simulink model "Linearhopf_squaretorque_0_5"  (R2019b)
settings: Solver=ode45  StartTime=0.0  StopTime=10  MaxStep=1e-3  RelTol=1e-3  AbsTol=1e-3
model workspace: external: MATLAB File sm_bumper_car_parameters.m (data not in the file)
undefined symbols (not defined in the file): BackLeft, BackRight, car, critical_velocity, damping, FrontLeft, FrontRight, g, kinetic_friction_coef, Link1, Link2, Link3, Link4, Link5, Link6, Link7, Link8, Link9, static_friction_coef, stiffness, transition_region_width, Wheel5, Wheel6, Wheel7, Wheel8, Wheel9, X, Y, Z
libraries: sm_lib x74, nesl_utility x19, sm_bumper_car_lib x9, simulink x7
(part 1 of 2)
Description:
  | Using the Spatial Contact Force Block - Bumper Car
settings Model: Creator=MathWorks  LastModifiedBy=hellomisscao
settings SolverCC: AutoScaleAbsTol=off
settings DataIOCC: ReturnWorkspaceOutputs=off
settings DebuggingCC: SymbolicDimsDataTypeCodeGenerationDiagnostic=none
settings SimscapeCC: SimscapeLogType=all  SimscapeLogSimulationStatistics=on  SimscapeLogName=simlog_sm_bumper_car  SimscapeLogDataHistory=20000
settings ExplorerConfigSet: InternalSimMechanicsExplorerSettings="<ExplorerConfiguration><canonicalview>default</canonicalview><AnimationSetting><BasePlaybackSpeed>1.0</BasePlaybackSpeed><PlaybackSpeedFactor>1.0</PlaybackSpeedFactor></AnimationSetting><TilePanel><TileInfo><Tiles Columns=\"1\" Count=\"1\" Rows=\"1\"><Column Weight=\"1\"/><Row Weight=\"1\"/><Tile Height=\"1\" Width=\"1\" X=\"0\" Y=\"0\"/></Tiles></TileInfo><SceneInfo><SceneViewer><BGColor><R>0.800000011920928955</R><G>0.800000011920928955</G><B>0.800000011920928955</B></BGColor><Camera><DoPerspective>off</DoPerspective><Position><X>0.637508295609907183</X><Y>-0.637508296451667844</Y><Z>1.11601012334107264</Z></Position><Center><X>-0.00639254054797280813</X><Y>0.00639253970621195267</Y><Z>0.472109287183192672</Z></Center><Up><X>-0.408248290463863073</X><Y>0.408248290463863073</Y><Z>0.816496580927726145</Z></Up><ViewLimDist>1</ViewLimDist><YLim>0.759088869094848628</YLim><XLim>0.995304530142192112</XLim></Camera></SceneViewer></SceneInfo></TilePanel><MechEditorPanel><Cameras/><GfxPanelCameraMap/><VideoCreator><PlaybackSpeedRatio>1.0</PlaybackSpeedRatio><FrameRate>30</FrameRate><VideoFormat>Motion JPEG AVI</VideoFormat><FrameSize>auto</FrameSize></VideoCreator></MechEditorPanel></ExplorerConfiguration>"

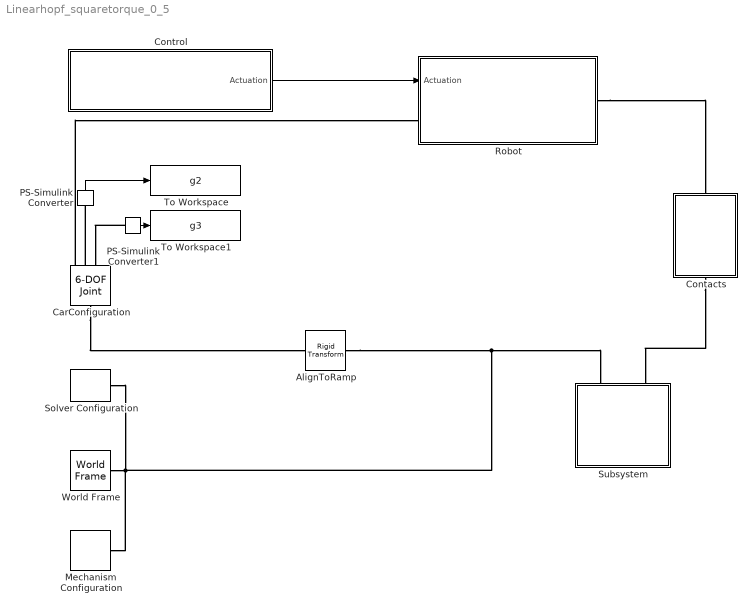
== system Linearhopf_squaretorque_0_5 ==
  AlignToRamp : sm_lib/Frames and Transforms/Rigid Transform  TranslationMethod=StandardAxis  TranslationStandardOffset=50 + 2*car.wheel.radius + 1  TranslationLengthUnit=cm  TranslationStandardAxis=+Z  TranslationCartesianOffset=[0 0 0]  TranslationROffset=0  TranslationROffsetUnits=m  TranslationZOffset=0  TranslationZOffsetUnits=m  TranslationThetaOffset=0  TranslationThetaOffsetUnits=deg  RotationMethod=StandardAxis  RotationAngleUnits=deg  RotationStandardAxis=+Y  RotationAngle=0  RotationArbitraryAxis=[0 0 1]  FollAlignAxisA=+X  BaseAlignAxisA=+Y  FollAlignAxisB=+Y  BaseAlignAxisB=+Z  RotationSequenceAxes=FollowerAxes  RotationSequence=XYX  RotationSequenceAngles=[0 0 0]  RotationSequenceAnglesUnits=deg  RotationMatrix=[1 0 0; 0 1 0; 0 0 1]
  CarConfiguration : sm_lib/Joints/6-DOF Joint  JointMode=Normal  SenseConstraintForce=off  SenseConstraintForceX=off  SenseConstraintForceY=off  SenseConstraintForceZ=off  SenseConstraintTorque=off  SenseConstraintTorqueX=off  SenseConstraintTorqueY=off  SenseConstraintTorqueZ=off  SenseTotalForce=off  SenseTotalForceX=off  SenseTotalForceY=off  SenseTotalForceZ=off  SenseTotalTorque=off  SenseTotalTorqueX=off  SenseTotalTorqueY=off  SenseTotalTorqueZ=off  CompositeWrenchDir=FollowerOnBase  CompositeWrenchFrame=BaseFrame  PxEquilibriumPosition=0  PxEquilibriumPositionUnits=m  PxSpringStiffness=0  PxSpringStiffnessUnits=N/m  PxDampingCoefficient=0  PxDampingCoefficientUnits=N/(m/s)  PxTorqueActuationMode=NoTorque  PxMotionActuationMode=ComputedMotion  PxSensePosition=on  PxSenseVelocity=off  PxSenseAcceleration=off  PxSenseTorqueForce=off  PxSenseLowerLimitTorqueForce=off  PxSenseUpperLimitTorqueForce=off  PxLowerLimitSpecify=off  PxLowerLimitBound=-1  PxLowerLimitBoundUnits=m  PxLowerLimitStiffness=1e6  PxLowerLimitStiffnessUnits=N/m  PxLowerLimitDamping=1e3  PxLowerLimitDampingUnits=N/(m/s)  PxLowerLimitTransitionRegionWidth=1e-4  PxLowerLimitTransitionRegionWidthUnits=m  PxUpperLimitSpecify=off  PxUpperLimitBound=1  PxUpperLimitBoundUnits=m  PxUpperLimitStiffness=1e6  PxUpperLimitStiffnessUnits=N/m  PxUpperLimitDamping=1e3  PxUpperLimitDampingUnits=N/(m/s)  PxUpperLimitTransitionRegionWidth=1e-4  PxUpperLimitTransitionRegionWidthUnits=m  PxPositionTargetSpecify=on  PxPositionTargetPriority=High  PxPositionTargetValue=car.start_dist  PxPositionTargetValueUnits=cm  PxVelocityTargetSpecify=off  PxVelocityTargetPriority=High  PxVelocityTargetValue=0  PxVelocityTargetValueUnits=m/s  PyEquilibriumPosition=0  PyEquilibriumPositionUnits=m  PySpringStiffness=0  PySpringStiffnessUnits=N/m  PyDampingCoefficient=0  PyDampingCoefficientUnits=N/(m/s)  PyTorqueActuationMode=NoTorque  PyMotionActuationMode=ComputedMotion  PySensePosition=on  PySenseVelocity=off  PySenseAcceleration=off  PySenseTorqueForce=off  PySenseLowerLimitTorqueForce=off  PySenseUpperLimitTorqueForce=off  PyLowerLimitSpecify=off  PyLowerLimitBound=-1  PyLowerLimitBoundUnits=m  PyLowerLimitStiffness=1e6  PyLowerLimitStiffnessUnits=N/m  PyLowerLimitDamping=1e3  PyLowerLimitDampingUnits=N/(m/s)  PyLowerLimitTransitionRegionWidth=1e-4  PyLowerLimitTransitionRegionWidthUnits=m  PyUpperLimitSpecify=off  PyUpperLimitBound=1  PyUpperLimitBoundUnits=m  PyUpperLimitStiffness=1e6  PyUpperLimitStiffnessUnits=N/m  PyUpperLimitDamping=1e3  PyUpperLimitDampingUnits=N/(m/s)  PyUpperLimitTransitionRegionWidth=1e-4  PyUpperLimitTransitionRegionWidthUnits=m  PyPositionTargetSpecify=off  PyPositionTargetPriority=High  PyPositionTargetValue=0  PyPositionTargetValueUnits=m  PyVelocityTargetSpecify=off  PyVelocityTargetPriority=High  PyVelocityTargetValue=0  PyVelocityTargetValueUnits=m/s  PzEquilibriumPosition=0  PzEquilibriumPositionUnits=m  PzSpringStiffness=0  PzSpringStiffnessUnits=N/m  PzDampingCoefficient=0  PzDampingCoefficientUnits=N/(m/s)  PzTorqueActuationMode=NoTorque  PzMotionActuationMode=ComputedMotion  PzSensePosition=on  PzSenseVelocity=off  PzSenseAcceleration=off  PzSenseTorqueForce=off  PzSenseLowerLimitTorqueForce=off  PzSenseUpperLimitTorqueForce=off  PzLowerLimitSpecify=off  PzLowerLimitBound=-1  PzLowerLimitBoundUnits=m  PzLowerLimitStiffness=1e6  PzLowerLimitStiffnessUnits=N/m  PzLowerLimitDamping=1e3  PzLowerLimitDampingUnits=N/(m/s)  PzLowerLimitTransitionRegionWidth=1e-4  PzLowerLimitTransitionRegionWidthUnits=m  PzUpperLimitSpecify=off  PzUpperLimitBound=1  PzUpperLimitBoundUnits=m  PzUpperLimitStiffness=1e6  PzUpperLimitStiffnessUnits=N/m  PzUpperLimitDamping=1e3  PzUpperLimitDampingUnits=N/(m/s)  PzUpperLimitTransitionRegionWidth=1e-4  PzUpperLimitTransitionRegionWidthUnits=m  PzPositionTargetSpecify=on  PzPositionTargetPriority=High  PzPositionTargetValue=car.start_height  PzPositionTargetValueUnits=cm  PzVelocityTargetSpecify=off  PzVelocityTargetPriority=High  PzVelocityTargetValue=0  PzVelocityTargetValueUnits=m/s  SphDefPosRotationMethod=None  SphDefPosRotationAngleUnits=deg  SphDefPosRotationStandardAxis=+Z  SphDefPosRotationAngle=0.0  SphDefPosRotationArbitraryAxis=[0 0 1]  SphDefPosFollAlignAxisA=+X  SphDefPosBaseAlignAxisA=+Y  SphDefPosFollAlignAxisB=+Y  SphDefPosBaseAlignAxisB=+Z  SphDefPosRotationSequenceAxes=FollowerAxes  SphDefPosRotationSequence=XYX  SphDefPosRotationSequenceAngles=[0 0 0]  SphDefPosRotationSequenceAnglesUnits=deg  SphDefPosRotationMatrix=[1 0 0; 0 1 0; 0 0 1]  SphEqPosRotationMethod=None  SphEqPosRotationAngleUnits=deg  SphEqPosRotationStandardAxis=+Z  SphEqPosRotationAngle=0.0  SphEqPosRotationArbitraryAxis=[0 0 1]  SphEqPosFollAlignAxisA=+X  SphEqPosBaseAlignAxisA=+Y  SphEqPosFollAlignAxisB=+Y  SphEqPosBaseAlignAxisB=+Z  SphEqPosRotationSequenceAxes=FollowerAxes  SphEqPosRotationSequence=XYX  SphEqPosRotationSequenceAngles=[0 0 0]  SphEqPosRotationSequenceAnglesUnits=deg  SphEqPosRotationMatrix=[1 0 0; 0 1 0; 0 0 1]  SphSpringStiffness=0  SphSpringStiffnessUnits=N*m/deg  SphDampingCoefficient=0  SphDampingCoefficientUnits=N*m/(deg/s)  SphActuateTorqueX=off  SphActuateTorqueY=off  SphActuateTorqueZ=off  SphActuateTorque=off  SphTorqueActuationMode=NoTorque  SphMotionActuationMode=ComputedMotion  SphActuationFrame=BaseFrame  SphSensePosition=off  SphSenseVelocityX=off  SphSenseVelocityY=off  SphSenseVelocityZ=off  SphSenseVelocity=off  SphSenseAccelerationX=off  SphSenseAccelerationY=off  SphSenseAccelerationZ=off  SphSenseAcceleration=off  SphSenseTorqueX=off  SphSenseTorqueY=off  SphSenseTorqueZ=off  SphSenseTorqueForce=off  SphSenseLowerLimitTorqueMag=off  SphSenseUpperLimitTorqueMag=off  SphSensingFrame=BaseFrame  SphLowerLimitSpecify=off  SphLowerLimitBound=15  SphLowerLimitBoundUnits=deg  SphLowerLimitStiffness=1e4  SphLowerLimitStiffnessUnits=N*m/deg  SphLowerLimitDamping=10  SphLowerLimitDampingUnits=N*m/(deg/s)  SphLowerLimitTransitionRegionWidth=0.1  SphLowerLimitTransitionRegionWidthUnits=deg  SphUpperLimitSpecify=off  SphUpperLimitBound=45  SphUpperLimitBoundUnits=deg  SphUpperLimitStiffness=1e4  SphUpperLimitStiffnessUnits=N*m/deg  SphUpperLimitDamping=10  SphUpperLimitDampingUnits=N*m/(deg/s)  SphUpperLimitTransitionRegionWidth=0.1  SphUpperLimitTransitionRegionWidthUnits=deg  SphPositionTargetRotationMethod=StandardAxis  SphPositionTargetRotationAngleUnits=deg  SphPositionTargetRotationStandardAxis=-Y  SphPositionTargetRotationAngle=car.start_pitch  SphPositionTargetRotationArbitraryAxis=[0 0 1]  SphPositionTargetFollAlignAxisA=+X  SphPositionTargetBaseAlignAxisA=+Y  SphPositionTargetFollAlignAxisB=+Y  SphPositionTargetBaseAlignAxisB=+Z  SphPositionTargetRotationSequenceAxes=FollowerAxes  SphPositionTargetRotationSequence=XYX  SphPositionTargetRotationSequenceAngles=[0 0 0]  SphPositionTargetRotationSequenceAnglesUnits=deg  SphPositionTargetRotationMatrix=[1 0 0; 0 1 0; 0 0 1]  SphPositionTargetSpecify=off  SphPositionTargetPriority=High  SphVelocityTargetValue=[0 0 0]  SphVelocityTargetValueUnits=deg/s  SphVelocityTargetSpecify=off  SphVelocityTargetPriority=High  SphVelocityTargetInFollowerFrame=on
  Contacts : Subsystem  mask{k=stiffness, b=damping, tau=transition_region_width, mus=static_friction_coef, muk=kinetic_friction_coef, cv=critical_velocity}
      mask prompts: k "Stiffness (N/m)"; b "Damping (N/(m/s))"; tau "Transition Region Width (m)"; mus "Coefficient of Static Friction"; muk "Coefficient of Kinetic Friction"; cv "Critical Velocity (m/s)"
  Control : Subsystem
  Mechanism Configuration : sm_lib/Utilities/Mechanism Configuration  UniformGravity=Constant  GravityVector=[0 0 -g]  GravityUnits=m/s^2  LinearizationDelta=0.001
  PS-Simulink Converter : nesl_utility/PS-Simulink Converter  PhysicalDomain=network_engine_domain  SubClassName=ps_output  LeftPortType=input  RightPortType=output  PseudoPeriodic=off  Frequencies=[]  Unit=inherit  AffineConversion=off
  PS-Simulink Converter1 : nesl_utility/PS-Simulink Converter  PhysicalDomain=network_engine_domain  SubClassName=ps_output  LeftPortType=input  RightPortType=output  PseudoPeriodic=off  Frequencies=[]  Unit=inherit  AffineConversion=off
  Robot : Subsystem  mask{l=car.body.length, w=car.body.width, h=car.body.height, m=car.body.mass, body_color=car.body.color, wheel_radius=car.wheel.radius, wheel_width=car.wheel.thickness, wheel_m=car.wheel.mass, wheel_color=car.wheel.color, wheel_spoke_color=car.wheel.spoke.color}
      mask prompts: l "Length (cm)"; w "Width (cm)"; h "Height (cm)"; m "Body Mass (kg)"; body_color "Car Body Color"; wheel_radius "Radius"; wheel_width "Thickness"; wheel_m "Wheel Mass (kg)"; wheel_color "Wheel Color"; wheel_spoke_color "Wheel Spoke Color"
      mask init:
      | axle_len               = .85 * l;
      | axle_radius            = axle_len / 30;
      | wheel_inner_radius     = .67 * wheel_radius;
      | wheel_spoke_thickness = axle_radius / 2;
      | 
      | front_wheel_pos  = l * .12;
      | back_wheel_pos   = l * .88;
      | wheel_separation = axle_len;
      mask DialogControl BodyGroupVar Prompt: Body
      mask DialogControl BodyDimGroupVar Prompt: Dimensions
      mask DialogControl BodyInertiaGroupVar Prompt: Inertia
      mask DialogControl BodyGraphicGroupVar Prompt: Graphic
      mask DialogControl WheelGroupVar Prompt: Wheels
      mask DialogControl WheelDimGroupVar Prompt: Dimensions
      mask DialogControl WheelInertiaGroupVar Prompt: Inertia
      mask DialogControl WheelGraphicGroupVar Prompt: Graphic
      mask Display: image('$imagefile'); % Use "Edit Image" on toolstrip to change.
  Solver Configuration : nesl_utility/Solver Configuration  PhysicalDomain=network_engine_domain  SubClassName=solver  LeftPortType=input  RightPortType=generic  Tones=[]  Harmonics=[]  SimulateNoise=off  Profile=off  UseLocalSampling=off  EnableSwitchedLinearOptims=on  FrequencyDomain=off  UseCCode=off  RelTol=0.001  AbsTol=1e-06  MinStep=1e-09  ToWorkspace=off  RevertToSquareIcSolve=off  NumHomotopyIterations=100  PhasorMode=off  PhasorModeNumHarmonics=1  DoDC=off  ResidualTolerance=1e-09  UseLocalSolver=off  LocalSolverChoice=NE_BACKWARD_EULER_ADVANCER  LocalSolverSampleTime=0.001  DoFixedCost=off  MaxNonlinIter=3  MaxModeIter=2  LinearAlgebra=Sparse  EquationFormulation=NE_TIME_EF  DelaysMemoryBudget=1024  AutomaticFiltering=on  FilteringTimeConstant=0.001  PartitionStorageMethod=AS_NEEDED  PartitionMemoryBudget=1024  PartitionMethod=FAST
  Subsystem : Subsystem
  To Workspace : ToWorkspace  VariableName=g2  SampleTime=-1
  To Workspace1 : ToWorkspace  VariableName=g3  SampleTime=-1
  World Frame : sm_lib/Frames and Transforms/World Frame
  wires:
  Control/1(Actuation) -> Robot/1(Actuation)
  PS-Simulink Converter/1 -> To Workspace/1
  PS-Simulink Converter1/1 -> To Workspace1/1
  connections:
  CarConfiguration/RConn1 -- Robot/LConn1
  Solver Configuration/RConn1 -- Mechanism Configuration/RConn1 -- Subsystem/RConn1 -- AlignToRamp/LConn1 -- World Frame/RConn1
  Robot/RConn1 -- Contacts/RConn1
  Contacts/LConn1 -- Subsystem/RConn2
  CarConfiguration/LConn1 -- AlignToRamp/RConn1
  CarConfiguration/RConn2 -- PS-Simulink Converter/LConn1
  PS-Simulink Converter1/LConn1 -- CarConfiguration/RConn3

== system Linearhopf_squaretorque_0_5/Contacts ==
  Car to Ramp 1 : Subsystem
  Ramps : PMIOPort  Side=Left
  Car : PMIOPort  Port=2  Side=Right
  connections:
  Car/RConn1 -- Car to Ramp 1/RConn1
  Ramps/RConn1 -- Car to Ramp 1/LConn1

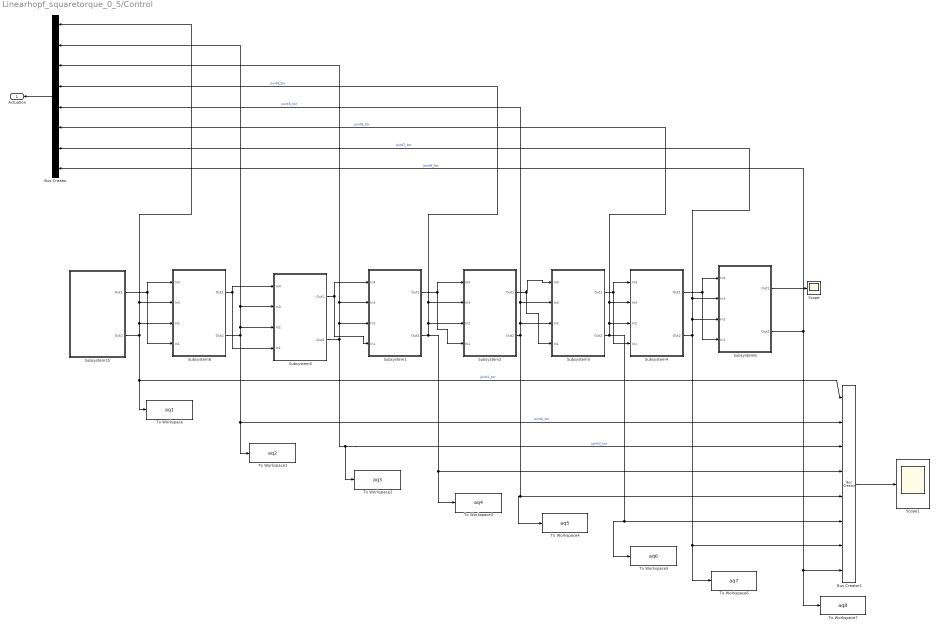
== system Linearhopf_squaretorque_0_5/Control ==
  Bus Creator : BusCreator  Inputs=8
  Bus Creator1 : BusCreator  Inputs=8
  Scope : Scope
  Scope1 : Scope
  Subsystem1 : Subsystem
  Subsystem15 : Subsystem
  Subsystem2 : Subsystem
  Subsystem3 : Subsystem
  Subsystem4 : Subsystem
  Subsystem5 : Subsystem
  Subsystem6 : Subsystem
  Subsystem8 : Subsystem
  To Workspace : ToWorkspace  VariableName=aq1  SaveFormat=Timeseries  SampleTime=-1
  To Workspace1 : ToWorkspace  VariableName=aq2  SaveFormat=Timeseries  SampleTime=-1
  To Workspace2 : ToWorkspace  VariableName=aq3  SaveFormat=Timeseries  SampleTime=-1
  To Workspace3 : ToWorkspace  VariableName=aq4  SaveFormat=Timeseries  SampleTime=-1
  To Workspace4 : ToWorkspace  VariableName=aq5  SaveFormat=Timeseries  SampleTime=-1
  To Workspace5 : ToWorkspace  VariableName=aq6  SaveFormat=Timeseries  SampleTime=-1
  To Workspace6 : ToWorkspace  VariableName=aq7  SaveFormat=Timeseries  SampleTime=-1
  To Workspace7 : ToWorkspace  VariableName=aq8  SaveFormat=Timeseries  SampleTime=-1
  Actuation : Outport
  wires:
  Subsystem5/2(Out2) -> Subsystem1/3(In2), Subsystem1/2(In3), Bus Creator/3, Bus Creator1/3, To Workspace2/1  "joint3_tor"
  Subsystem3/2(Out2) -> Subsystem4/3(In2), Bus Creator/6, Subsystem4/2(In3), To Workspace5/1, Bus Creator1/6  "joint6_tor"
  Subsystem8/2(Out2) -> Bus Creator/2, Subsystem5/2(In3), Subsystem5/3(In2), Bus Creator1/2, To Workspace1/1  "joint2_tor"
  Bus Creator/1 -> Actuation/1
  Subsystem1/2(Out2) -> To Workspace3/1, Bus Creator1/4, Subsystem2/2(In3), Bus Creator/4, Subsystem2/3(In2)  "joint4_tor"
  Subsystem4/2(Out2) -> To Workspace6/1, Bus Creator1/7, Subsystem6/3(In2), Bus Creator/7, Subsystem6/2(In3)  "joint7_tor"
  Subsystem6/2(Out2) -> To Workspace7/1, Bus Creator1/8, Bus Creator/8  "joint8_tor"
  Subsystem2/2(Out2) -> Subsystem3/3(In2), Bus Creator/5, Subsystem3/2(In3), To Workspace4/1, Bus Creator1/5  "joint5_tor"
  Subsystem15/2(Out2) -> To Workspace/1, Bus Creator1/1, Subsystem8/2(In3), Bus Creator/1, Subsystem8/3(In2)  "joint1_tor"
  Subsystem4/1(Out1) -> Subsystem6/1(In4), Subsystem6/4(In1)
  Subsystem3/1(Out1) -> Subsystem4/1(In4), Subsystem4/4(In1)
  Subsystem15/1(Out1) -> Subsystem8/4(In1), Subsystem8/1(In4)
  Subsystem1/1(Out1) -> Subsystem2/4(In1), Subsystem2/1(In4)
  Subsystem6/1(Out1) -> Scope/1
  Bus Creator1/1 -> Scope1/1
  Subsystem8/1(Out1) -> Subsystem5/4(In1), Subsystem5/1(In4)
  Subsystem5/1(Out1) -> Subsystem1/1(In4), Subsystem1/4(In1)
  Subsystem2/1(Out1) -> Subsystem3/1(In4), Subsystem3/4(In1)

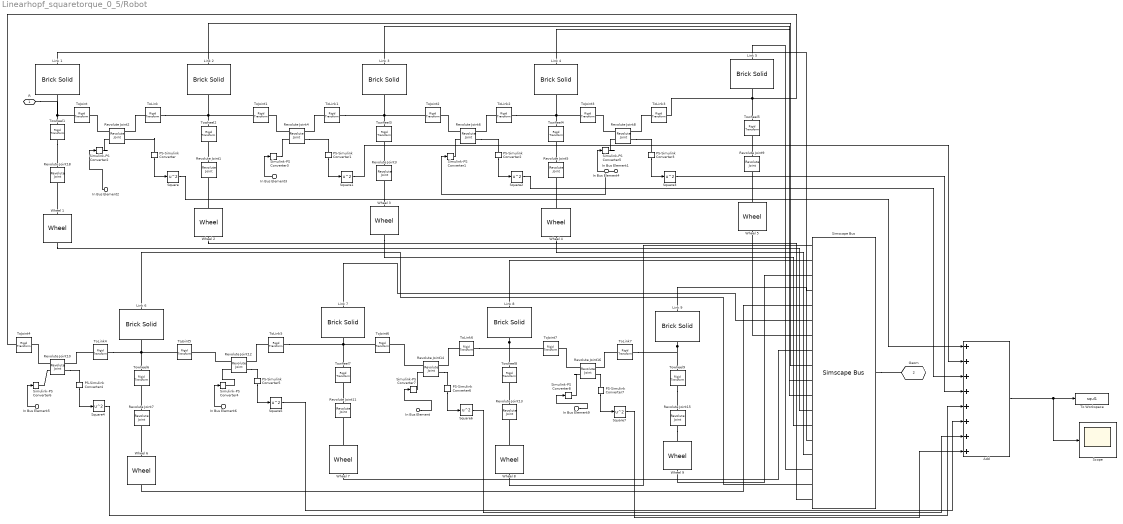
== system Linearhopf_squaretorque_0_5/Robot ==
  In Bus Element2 : Inport  PortName=Actuation  Element=joint1_tor
  In Bus Element3 : Inport  PortName=Actuation  Element=joint2_tor
  In Bus Element1 : Inport  PortName=Actuation  Element=joint3_tor
  In Bus Element4 : Inport  PortName=Actuation  Element=joint4_tor
  In Bus Element5 : Inport  PortName=Actuation  Element=joint5_tor
  In Bus Element6 : Inport  PortName=Actuation  Element=joint6_tor
  In Bus Element : Inport  PortName=Actuation  Element=joint7_tor
  In Bus Element9 : Inport  PortName=Actuation  Element=joint8_tor
  Add : Sum  Inputs=++++++++
  Link 1 : sm_lib/Body Elements/Brick Solid  GraphicAmbientColor=[0.15 0.15 0.15 1.0]  BasedOnType=Mass  BrickDimensions=[l w h]  BrickDimensionUnits=cm  CenterOfMass=[0 0 0]  CenterOfMassUnits=cm  GraphicDiffuseColor=[0.8 0.8 0.0]  Density=1000  DensityUnits=kg/m^3  DoExposeReferenceFrame=on  GraphicEmissiveColor=[0.0 0.0 0.0 1.0]  ExportEntireGeometry=on  SerializedFrames=<Frames/>  MarkerShape=Sphere  MarkerSize=10  GraphicType=FromGeometry  InertiaType=CalculateFromGeometry  Mass=m  MassUnits=kg  MomentsOfInertia=[1 1 1]  MomentsOfInertiaUnits=kg*m^2  GraphicOpacity=1.0  ProductsOfInertia=[0 0 0]  ProductsOfInertiaUnits=kg*m^2  GraphicShininess=75  GraphicSpecularColor=[0.5 0.5 0.5 1.0]  GraphicVisPropType=SimpleVisualProperties
  Link {2..9} (8 alike) : sm_lib/Body Elements/Brick Solid  GraphicAmbientColor=[0.15 0.15 0.15 1.0]  BasedOnType=Mass  BrickDimensions=[l w h]  BrickDimensionUnits=cm  CenterOfMass=[0 0 0]  CenterOfMassUnits=cm  GraphicDiffuseColor=[1.0 0.2 0.0]  Density=1000  DensityUnits=kg/m^3  DoExposeReferenceFrame=on  GraphicEmissiveColor=[0.0 0.0 0.0 1.0]  ExportEntireGeometry=on  SerializedFrames=<Frames/>  MarkerShape=Sphere  MarkerSize=10  GraphicType=FromGeometry  InertiaType=CalculateFromGeometry  Mass=m  MassUnits=kg  MomentsOfInertia=[1 1 1]  MomentsOfInertiaUnits=kg*m^2  GraphicOpacity=1.0  ProductsOfInertia=[0 0 0]  ProductsOfInertiaUnits=kg*m^2  GraphicShininess=75  GraphicSpecularColor=[0.5 0.5 0.5 1.0]  GraphicVisPropType=SimpleVisualProperties
  PS-Simulink Converter{,1..7} (8 alike) : nesl_utility/PS-Simulink Converter  PhysicalDomain=network_engine_domain  SubClassName=ps_output  LeftPortType=input  RightPortType=output  PseudoPeriodic=off  Frequencies=[]  Unit=inherit  AffineConversion=off
  Revolute Joint{1,3,5,7,9,11,13,15,18} (9 alike) : sm_lib/Joints/Revolute Joint  JointMode=Normal  SenseConstraintForce=off  SenseConstraintForceX=off  SenseConstraintForceY=off  SenseConstraintForceZ=off  SenseConstraintTorque=off  SenseConstraintTorqueX=off  SenseConstraintTorqueY=off  SenseConstraintTorqueZ=off  SenseTotalForce=off  SenseTotalForceX=off  SenseTotalForceY=off  SenseTotalForceZ=off  SenseTotalTorque=off  SenseTotalTorqueX=off  SenseTotalTorqueY=off  SenseTotalTorqueZ=off  CompositeWrenchDir=FollowerOnBase  CompositeWrenchFrame=BaseFrame  EquilibriumPosition=0  EquilibriumPositionUnits=deg  SpringStiffness=0  SpringStiffnessUnits=N*m/deg  DampingCoefficient=0  DampingCoefficientUnits=N*m/(deg/s)  TorqueActuationMode=NoTorque  MotionActuationMode=ComputedMotion  SensePosition=off  SenseVelocity=off  SenseAcceleration=off  SenseTorqueForce=off  SenseLowerLimitTorqueForce=off  SenseUpperLimitTorqueForce=off  LowerLimitSpecify=off  LowerLimitBound=-90  LowerLimitBoundUnits=deg  LowerLimitStiffness=1e4  LowerLimitStiffnessUnits=N*m/deg  LowerLimitDamping=10  LowerLimitDampingUnits=N*m/(deg/s)  LowerLimitTransitionRegionWidth=0.1  LowerLimitTransitionRegionWidthUnits=deg  UpperLimitSpecify=off  UpperLimitBound=90  UpperLimitBoundUnits=deg  UpperLimitStiffness=1e4  UpperLimitStiffnessUnits=N*m/deg  UpperLimitDamping=10  UpperLimitDampingUnits=N*m/(deg/s)  UpperLimitTransitionRegionWidth=0.1  UpperLimitTransitionRegionWidthUnits=deg  PositionTargetSpecify=off  PositionTargetPriority=High  PositionTargetValue=0  PositionTargetValueUnits=deg  VelocityTargetSpecify=off  VelocityTargetPriority=High  VelocityTargetValue=0  VelocityTargetValueUnits=deg/s
  Revolute Joint10 : sm_lib/Joints/Revolute Joint  JointMode=Normal  SenseConstraintForce=off  SenseConstraintForceX=off  SenseConstraintForceY=off  SenseConstraintForceZ=off  SenseConstraintTorque=off  SenseConstraintTorqueX=off  SenseConstraintTorqueY=off  SenseConstraintTorqueZ=off  SenseTotalForce=off  SenseTotalForceX=off  SenseTotalForceY=off  SenseTotalForceZ=off  SenseTotalTorque=off  SenseTotalTorqueX=off  SenseTotalTorqueY=off  SenseTotalTorqueZ=off  CompositeWrenchDir=FollowerOnBase  CompositeWrenchFrame=BaseFrame  EquilibriumPosition=0  EquilibriumPositionUnits=deg  SpringStiffness=0.001  SpringStiffnessUnits=N*m/deg  DampingCoefficient=0  DampingCoefficientUnits=N*m/(deg/s)  TorqueActuationMode=ComputedTorque  MotionActuationMode=InputMotion  SensePosition=off  SenseVelocity=off  SenseAcceleration=off  SenseTorqueForce=on  SenseLowerLimitTorqueForce=off  SenseUpperLimitTorqueForce=off  LowerLimitSpecify=off  LowerLimitBound=-90  LowerLimitBoundUnits=deg  LowerLimitStiffness=1e4  LowerLimitStiffnessUnits=N*m/deg  LowerLimitDamping=10  LowerLimitDampingUnits=N*m/(deg/s)  LowerLimitTransitionRegionWidth=0.1  LowerLimitTransitionRegionWidthUnits=deg  UpperLimitSpecify=off  UpperLimitBound=90  UpperLimitBoundUnits=deg  UpperLimitStiffness=1e4  UpperLimitStiffnessUnits=N*m/deg  UpperLimitDamping=10  UpperLimitDampingUnits=N*m/(deg/s)  UpperLimitTransitionRegionWidth=0.1  UpperLimitTransitionRegionWidthUnits=deg  PositionTargetSpecify=on  PositionTargetPriority=High  PositionTargetValue=-0.05  PositionTargetValueUnits=rad  VelocityTargetSpecify=off  VelocityTargetPriority=High  VelocityTargetValue=0  VelocityTargetValueUnits=deg/s
  Revolute Joint12 : sm_lib/Joints/Revolute Joint  JointMode=Normal  SenseConstraintForce=off  SenseConstraintForceX=off  SenseConstraintForceY=off  SenseConstraintForceZ=off  SenseConstraintTorque=off  SenseConstraintTorqueX=off  SenseConstraintTorqueY=off  SenseConstraintTorqueZ=off  SenseTotalForce=off  SenseTotalForceX=off  SenseTotalForceY=off  SenseTotalForceZ=off  SenseTotalTorque=off  SenseTotalTorqueX=off  SenseTotalTorqueY=off  SenseTotalTorqueZ=off  CompositeWrenchDir=FollowerOnBase  CompositeWrenchFrame=BaseFrame  EquilibriumPosition=0  EquilibriumPositionUnits=deg  SpringStiffness=0.001  SpringStiffnessUnits=N*m/deg  DampingCoefficient=0  DampingCoefficientUnits=N*m/(deg/s)  TorqueActuationMode=ComputedTorque  MotionActuationMode=InputMotion  SensePosition=off  SenseVelocity=off  SenseAcceleration=off  SenseTorqueForce=on  SenseLowerLimitTorqueForce=off  SenseUpperLimitTorqueForce=off  LowerLimitSpecify=off  LowerLimitBound=-90  LowerLimitBoundUnits=deg  LowerLimitStiffness=1e4  LowerLimitStiffnessUnits=N*m/deg  LowerLimitDamping=10  LowerLimitDampingUnits=N*m/(deg/s)  LowerLimitTransitionRegionWidth=0.1  LowerLimitTransitionRegionWidthUnits=deg  UpperLimitSpecify=off  UpperLimitBound=90  UpperLimitBoundUnits=deg  UpperLimitStiffness=1e4  UpperLimitStiffnessUnits=N*m/deg  UpperLimitDamping=10  UpperLimitDampingUnits=N*m/(deg/s)  UpperLimitTransitionRegionWidth=0.1  UpperLimitTransitionRegionWidthUnits=deg  PositionTargetSpecify=on  PositionTargetPriority=High  PositionTargetValue=-0.1  PositionTargetValueUnits=rad  VelocityTargetSpecify=off  VelocityTargetPriority=High  VelocityTargetValue=0  VelocityTargetValueUnits=deg/s
  Revolute Joint14 : sm_lib/Joints/Revolute Joint  JointMode=Normal  SenseConstraintForce=off  SenseConstraintForceX=off  SenseConstraintForceY=off  SenseConstraintForceZ=off  SenseConstraintTorque=off  SenseConstraintTorqueX=off  SenseConstraintTorqueY=off  SenseConstraintTorqueZ=off  SenseTotalForce=off  SenseTotalForceX=off  SenseTotalForceY=off  SenseTotalForceZ=off  SenseTotalTorque=off  SenseTotalTorqueX=off  SenseTotalTorqueY=off  SenseTotalTorqueZ=off  CompositeWrenchDir=FollowerOnBase  CompositeWrenchFrame=BaseFrame  EquilibriumPosition=0  EquilibriumPositionUnits=deg  SpringStiffness=0.001  SpringStiffnessUnits=N*m/deg  DampingCoefficient=0  DampingCoefficientUnits=N*m/(deg/s)  TorqueActuationMode=ComputedTorque  MotionActuationMode=InputMotion  SensePosition=off  SenseVelocity=off  SenseAcceleration=off  SenseTorqueForce=on  SenseLowerLimitTorqueForce=off  SenseUpperLimitTorqueForce=off  LowerLimitSpecify=off  LowerLimitBound=-90  LowerLimitBoundUnits=deg  LowerLimitStiffness=1e4  LowerLimitStiffnessUnits=N*m/deg  LowerLimitDamping=10  LowerLimitDampingUnits=N*m/(deg/s)  LowerLimitTransitionRegionWidth=0.1  LowerLimitTransitionRegionWidthUnits=deg  UpperLimitSpecify=off  UpperLimitBound=90  UpperLimitBoundUnits=deg  UpperLimitStiffness=1e4  UpperLimitStiffnessUnits=N*m/deg  UpperLimitDamping=10  UpperLimitDampingUnits=N*m/(deg/s)  UpperLimitTransitionRegionWidth=0.1  UpperLimitTransitionRegionWidthUnits=deg  PositionTargetSpecify=on  PositionTargetPriority=High  PositionTargetValue=-0.05  PositionTargetValueUnits=rad  VelocityTargetSpecify=off  VelocityTargetPriority=High  VelocityTargetValue=0  VelocityTargetValueUnits=deg/s
  Revolute Joint16 : sm_lib/Joints/Revolute Joint  JointMode=Normal  SenseConstraintForce=off  SenseConstraintForceX=off  SenseConstraintForceY=off  SenseConstraintForceZ=off  SenseConstraintTorque=off  SenseConstraintTorqueX=off  SenseConstraintTorqueY=off  SenseConstraintTorqueZ=off  SenseTotalForce=off  SenseTotalForceX=off  SenseTotalForceY=off  SenseTotalForceZ=off  SenseTotalTorque=off  SenseTotalTorqueX=off  SenseTotalTorqueY=off  SenseTotalTorqueZ=off  CompositeWrenchDir=FollowerOnBase  CompositeWrenchFrame=BaseFrame  EquilibriumPosition=0  EquilibriumPositionUnits=deg  SpringStiffness=0.001  SpringStiffnessUnits=N*m/deg  DampingCoefficient=0  DampingCoefficientUnits=N*m/(deg/s)  TorqueActuationMode=ComputedTorque  MotionActuationMode=InputMotion  SensePosition=off  SenseVelocity=off  SenseAcceleration=off  SenseTorqueForce=on  SenseLowerLimitTorqueForce=off  SenseUpperLimitTorqueForce=off  LowerLimitSpecify=off  LowerLimitBound=-90  LowerLimitBoundUnits=deg  LowerLimitStiffness=1e4  LowerLimitStiffnessUnits=N*m/deg  LowerLimitDamping=10  LowerLimitDampingUnits=N*m/(deg/s)  LowerLimitTransitionRegionWidth=0.1  LowerLimitTransitionRegionWidthUnits=deg  UpperLimitSpecify=off  UpperLimitBound=90  UpperLimitBoundUnits=deg  UpperLimitStiffness=1e4  UpperLimitStiffnessUnits=N*m/deg  UpperLimitDamping=10  UpperLimitDampingUnits=N*m/(deg/s)  UpperLimitTransitionRegionWidth=0.1  UpperLimitTransitionRegionWidthUnits=deg  PositionTargetSpecify=on  PositionTargetPriority=High  PositionTargetValue=0  PositionTargetValueUnits=rad  VelocityTargetSpecify=off  VelocityTargetPriority=High  VelocityTargetValue=0  VelocityTargetValueUnits=deg/s
  Revolute Joint2 : sm_lib/Joints/Revolute Joint  JointMode=Normal  SenseConstraintForce=off  SenseConstraintForceX=off  SenseConstraintForceY=off  SenseConstraintForceZ=off  SenseConstraintTorque=off  SenseConstraintTorqueX=off  SenseConstraintTorqueY=off  SenseConstraintTorqueZ=off  SenseTotalForce=off  SenseTotalForceX=off  SenseTotalForceY=off  SenseTotalForceZ=off  SenseTotalTorque=off  SenseTotalTorqueX=off  SenseTotalTorqueY=off  SenseTotalTorqueZ=off  CompositeWrenchDir=FollowerOnBase  CompositeWrenchFrame=BaseFrame  EquilibriumPosition=0  EquilibriumPositionUnits=deg  SpringStiffness=0.001  SpringStiffnessUnits=N*m/deg  DampingCoefficient=0  DampingCoefficientUnits=N*m/(deg/s)  TorqueActuationMode=ComputedTorque  MotionActuationMode=InputMotion  SensePosition=off  SenseVelocity=off  SenseAcceleration=off  SenseTorqueForce=on  SenseLowerLimitTorqueForce=off  SenseUpperLimitTorqueForce=off  LowerLimitSpecify=off  LowerLimitBound=-90  LowerLimitBoundUnits=deg  LowerLimitStiffness=1e4  LowerLimitStiffnessUnits=N*m/deg  LowerLimitDamping=10  LowerLimitDampingUnits=N*m/(deg/s)  LowerLimitTransitionRegionWidth=0.1  LowerLimitTransitionRegionWidthUnits=deg  UpperLimitSpecify=off  UpperLimitBound=90  UpperLimitBoundUnits=deg  UpperLimitStiffness=1e4  UpperLimitStiffnessUnits=N*m/deg  UpperLimitDamping=10  UpperLimitDampingUnits=N*m/(deg/s)  UpperLimitTransitionRegionWidth=0.1  UpperLimitTransitionRegionWidthUnits=deg  PositionTargetSpecify=on  PositionTargetPriority=High  PositionTargetValue=0.05  PositionTargetValueUnits=rad  VelocityTargetSpecify=off  VelocityTargetPriority=High  VelocityTargetValue=0  VelocityTargetValueUnits=deg/s
  Revolute Joint4 : sm_lib/Joints/Revolute Joint  JointMode=Normal  SenseConstraintForce=off  SenseConstraintForceX=off  SenseConstraintForceY=off  SenseConstraintForceZ=off  SenseConstraintTorque=off  SenseConstraintTorqueX=off  SenseConstraintTorqueY=off  SenseConstraintTorqueZ=off  SenseTotalForce=off  SenseTotalForceX=off  SenseTotalForceY=off  SenseTotalForceZ=off  SenseTotalTorque=off  SenseTotalTorqueX=off  SenseTotalTorqueY=off  SenseTotalTorqueZ=off  CompositeWrenchDir=FollowerOnBase  CompositeWrenchFrame=BaseFrame  EquilibriumPosition=0  EquilibriumPositionUnits=deg  SpringStiffness=0.001  SpringStiffnessUnits=N*m/deg  DampingCoefficient=0  DampingCoefficientUnits=N*m/(deg/s)  TorqueActuationMode=ComputedTorque  MotionActuationMode=InputMotion  SensePosition=off  SenseVelocity=off  SenseAcceleration=off  SenseTorqueForce=on  SenseLowerLimitTorqueForce=off  SenseUpperLimitTorqueForce=off  LowerLimitSpecify=off  LowerLimitBound=-90  LowerLimitBoundUnits=deg  LowerLimitStiffness=1e4  LowerLimitStiffnessUnits=N*m/deg  LowerLimitDamping=10  LowerLimitDampingUnits=N*m/(deg/s)  LowerLimitTransitionRegionWidth=0.1  LowerLimitTransitionRegionWidthUnits=deg  UpperLimitSpecify=off  UpperLimitBound=90  UpperLimitBoundUnits=deg  UpperLimitStiffness=1e4  UpperLimitStiffnessUnits=N*m/deg  UpperLimitDamping=10  UpperLimitDampingUnits=N*m/(deg/s)  UpperLimitTransitionRegionWidth=0.1  UpperLimitTransitionRegionWidthUnits=deg  PositionTargetSpecify=on  PositionTargetPriority=High  PositionTargetValue=0.1  PositionTargetValueUnits=rad  VelocityTargetSpecify=off  VelocityTargetPriority=High  VelocityTargetValue=0  VelocityTargetValueUnits=deg/s
  Revolute Joint6 : sm_lib/Joints/Revolute Joint  JointMode=Normal  SenseConstraintForce=off  SenseConstraintForceX=off  SenseConstraintForceY=off  SenseConstraintForceZ=off  SenseConstraintTorque=off  SenseConstraintTorqueX=off  SenseConstraintTorqueY=off  SenseConstraintTorqueZ=off  SenseTotalForce=off  SenseTotalForceX=off  SenseTotalForceY=off  SenseTotalForceZ=off  SenseTotalTorque=off  SenseTotalTorqueX=off  SenseTotalTorqueY=off  SenseTotalTorqueZ=off  CompositeWrenchDir=FollowerOnBase  CompositeWrenchFrame=BaseFrame  EquilibriumPosition=0  EquilibriumPositionUnits=deg  SpringStiffness=0.001  SpringStiffnessUnits=N*m/deg  DampingCoefficient=0  DampingCoefficientUnits=N*m/(deg/s)  TorqueActuationMode=ComputedTorque  MotionActuationMode=InputMotion  SensePosition=off  SenseVelocity=off  SenseAcceleration=off  SenseTorqueForce=on  SenseLowerLimitTorqueForce=off  SenseUpperLimitTorqueForce=off  LowerLimitSpecify=off  LowerLimitBound=-90  LowerLimitBoundUnits=deg  LowerLimitStiffness=1e4  LowerLimitStiffnessUnits=N*m/deg  LowerLimitDamping=10  LowerLimitDampingUnits=N*m/(deg/s)  LowerLimitTransitionRegionWidth=0.1  LowerLimitTransitionRegionWidthUnits=deg  UpperLimitSpecify=off  UpperLimitBound=90  UpperLimitBoundUnits=deg  UpperLimitStiffness=1e4  UpperLimitStiffnessUnits=N*m/deg  UpperLimitDamping=10  UpperLimitDampingUnits=N*m/(deg/s)  UpperLimitTransitionRegionWidth=0.1  UpperLimitTransitionRegionWidthUnits=deg  PositionTargetSpecify=on  PositionTargetPriority=High  PositionTargetValue=0.05  PositionTargetValueUnits=rad  VelocityTargetSpecify=off  VelocityTargetPriority=High  VelocityTargetValue=0  VelocityTargetValueUnits=deg/s
  Revolute Joint8 : sm_lib/Joints/Revolute Joint  JointMode=Normal  SenseConstraintForce=off  SenseConstraintForceX=off  SenseConstraintForceY=off  SenseConstraintForceZ=off  SenseConstraintTorque=off  SenseConstraintTorqueX=off  SenseConstraintTorqueY=off  SenseConstraintTorqueZ=off  SenseTotalForce=off  SenseTotalForceX=off  SenseTotalForceY=off  SenseTotalForceZ=off  SenseTotalTorque=off  SenseTotalTorqueX=off  SenseTotalTorqueY=off  SenseTotalTorqueZ=off  CompositeWrenchDir=FollowerOnBase  CompositeWrenchFrame=BaseFrame  EquilibriumPosition=0  EquilibriumPositionUnits=deg  SpringStiffness=0.001  SpringStiffnessUnits=N*m/deg  DampingCoefficient=0  DampingCoefficientUnits=N*m/(deg/s)  TorqueActuationMode=ComputedTorque  MotionActuationMode=InputMotion  SensePosition=off  SenseVelocity=off  SenseAcceleration=off  SenseTorqueForce=on  SenseLowerLimitTorqueForce=off  SenseUpperLimitTorqueForce=off  LowerLimitSpecify=off  LowerLimitBound=-90  LowerLimitBoundUnits=deg  LowerLimitStiffness=1e4  LowerLimitStiffnessUnits=N*m/deg  LowerLimitDamping=10  LowerLimitDampingUnits=N*m/(deg/s)  LowerLimitTransitionRegionWidth=0.1  LowerLimitTransitionRegionWidthUnits=deg  UpperLimitSpecify=off  UpperLimitBound=90  UpperLimitBoundUnits=deg  UpperLimitStiffness=1e4  UpperLimitStiffnessUnits=N*m/deg  UpperLimitDamping=10  UpperLimitDampingUnits=N*m/(deg/s)  UpperLimitTransitionRegionWidth=0.1  UpperLimitTransitionRegionWidthUnits=deg  PositionTargetSpecify=on  PositionTargetPriority=High  PositionTargetValue=0  PositionTargetValueUnits=rad  VelocityTargetSpecify=off  VelocityTargetPriority=High  VelocityTargetValue=0  VelocityTargetValueUnits=deg/s
  Scope : Scope
  Simscape Bus : SimscapeBus  HierarchyStrings=Wheel8;Link8;Wheel9;Link9;Wheel6;Link7;Wheel5;Wheel7;Link2;Link3;Link4;BackLeft;FrontLeft;Link1;FrontRight;Link5;Link6;BackRight
  Simulink-PS Converter{1..8} (8 alike) : nesl_utility/Simulink-PS Converter  PhysicalDomain=network_engine_domain  SubClassName=ps_input  LeftPortType=input  RightPortType=output  PseudoPeriodic=off  Frequencies=[]  NoiseDistribution=none  NoiseParameters=[]  Unit=1  AffineConversion=off  FilteringAndDerivatives=filter  SimscapeFilterOrder=2  InputFilterTimeConstant=0.01  UdotUserProvided=0
  Square{,1..7} (8 alike) : Math  Operator=square  SignedPower=off  SaturateOnIntegerOverflow=on
  To Workspace : ToWorkspace  VariableName=squl1  SaveFormat=Timeseries  SampleTime=-1
  ToJoint{,1..7} (8 alike) : sm_lib/Frames and Transforms/Rigid Transform  TranslationMethod=StandardAxis  TranslationStandardOffset=l /2 + 1  TranslationLengthUnit=cm  TranslationStandardAxis=+X  TranslationCartesianOffset=[0 0 0]  TranslationROffset=0  TranslationROffsetUnits=m  TranslationZOffset=0  TranslationZOffsetUnits=m  TranslationThetaOffset=0  TranslationThetaOffsetUnits=deg  RotationMethod=None  RotationAngleUnits=deg  RotationStandardAxis=+Z  RotationAngle=0.0  RotationArbitraryAxis=[0 0 1]  FollAlignAxisA=+Y  BaseAlignAxisA=+Z  FollAlignAxisB=+Z  BaseAlignAxisB=-Y  RotationSequenceAxes=FollowerAxes  RotationSequence=XYX  RotationSequenceAngles=[0 0 0]  RotationSequenceAnglesUnits=deg  RotationMatrix=[1 0 0; 0 1 0; 0 0 1]
  ToLink{,1..7} (8 alike) : sm_lib/Frames and Transforms/Rigid Transform  TranslationMethod=StandardAxis  TranslationStandardOffset=l /2 + 1  TranslationLengthUnit=cm  TranslationStandardAxis=+X  TranslationCartesianOffset=[0 0 0]  TranslationROffset=0  TranslationROffsetUnits=m  TranslationZOffset=0  TranslationZOffsetUnits=m  TranslationThetaOffset=0  TranslationThetaOffsetUnits=deg  RotationMethod=None  RotationAngleUnits=deg  RotationStandardAxis=+Z  RotationAngle=0.0  RotationArbitraryAxis=[0 0 1]  FollAlignAxisA=+Y  BaseAlignAxisA=+Z  FollAlignAxisB=+Z  BaseAlignAxisB=-Y  RotationSequenceAxes=FollowerAxes  RotationSequence=XYX  RotationSequenceAngles=[0 0 0]  RotationSequenceAnglesUnits=deg  RotationMatrix=[1 0 0; 0 1 0; 0 0 1]
  Towheel{1..9} (9 alike) : sm_lib/Frames and Transforms/Rigid Transform  TranslationMethod=StandardAxis  TranslationStandardOffset=h/2 + wheel_radius + 1  TranslationLengthUnit=cm  TranslationStandardAxis=-Z  TranslationCartesianOffset=[0 0 0]  TranslationROffset=0  TranslationROffsetUnits=m  TranslationZOffset=0  TranslationZOffsetUnits=m  TranslationThetaOffset=0  TranslationThetaOffsetUnits=deg  RotationMethod=AlignedAxes  RotationAngleUnits=deg  RotationStandardAxis=+Z  RotationAngle=0.0  RotationArbitraryAxis=[0 0 1]  FollAlignAxisA=+Y  BaseAlignAxisA=+Z  FollAlignAxisB=+Z  BaseAlignAxisB=-Y  RotationSequenceAxes=FollowerAxes  RotationSequence=XYX  RotationSequenceAngles=[0 0 0]  RotationSequenceAnglesUnits=deg  RotationMatrix=[1 0 0; 0 1 0; 0 0 1]
  Wheel 1 : sm_bumper_car_lib/Wheel  r=wheel_radius  rin=wheel_inner_radius  spoke_r=wheel_spoke_thickness  W=wheel_width  m=wheel_m  color=wheel_color  spoke_color=wheel_spoke_color
      link override Wheel Graphic: GraphicDiffuseColor=[0.2 0.2 0.2]
      settings: SourceProductBaseCode=MS
  Wheel 2 : sm_bumper_car_lib/Wheel  r=wheel_radius  rin=wheel_inner_radius  spoke_r=wheel_spoke_thickness  W=wheel_width  m=wheel_m  color=wheel_color  spoke_color=wheel_spoke_color
      link override Wheel Graphic: GraphicDiffuseColor=[0.2 0.2 0.2]
      settings: SourceProductBaseCode=MS
  Wheel 3 : sm_bumper_car_lib/Wheel  r=wheel_radius  rin=wheel_inner_radius  spoke_r=wheel_spoke_thickness  W=wheel_width  m=wheel_m  color=wheel_color  spoke_color=wheel_spoke_color
      link override Wheel Graphic: GraphicDiffuseColor=[0.2 0.2 0.2]
      settings: SourceProductBaseCode=MS
  Wheel 4 : sm_bumper_car_lib/Wheel  r=wheel_radius  rin=wheel_inner_radius  spoke_r=wheel_spoke_thickness  W=wheel_width  m=wheel_m  color=wheel_color  spoke_color=wheel_spoke_color
      link override Wheel Graphic: GraphicDiffuseColor=[0.2 0.2 0.2]
      settings: SourceProductBaseCode=MS
  Wheel 5 : sm_bumper_car_lib/Wheel  r=wheel_radius  rin=wheel_inner_radius  spoke_r=wheel_spoke_thickness  W=wheel_width  m=wheel_m  color=wheel_color  spoke_color=wheel_spoke_color
      link override Wheel Graphic: GraphicDiffuseColor=[0.2 0.2 0.2]
      settings: SourceProductBaseCode=MS
  Wheel 6 : sm_bumper_car_lib/Wheel  r=wheel_radius  rin=wheel_inner_radius  spoke_r=wheel_spoke_thickness  W=wheel_width  m=wheel_m  color=wheel_color  spoke_color=wheel_spoke_color
      link override Wheel Graphic: GraphicDiffuseColor=[0.2 0.2 0.2]
      settings: SourceProductBaseCode=MS
  Wheel 7 : sm_bumper_car_lib/Wheel  r=wheel_radius  rin=wheel_inner_radius  spoke_r=wheel_spoke_thickness  W=wheel_width  m=wheel_m  color=wheel_color  spoke_color=wheel_spoke_color
      link override Wheel Graphic: GraphicDiffuseColor=[0.2 0.2 0.2]
      settings: SourceProductBaseCode=MS
  Wheel 8 : sm_bumper_car_lib/Wheel  r=wheel_radius  rin=wheel_inner_radius  spoke_r=wheel_spoke_thickness  W=wheel_width  m=wheel_m  color=wheel_color  spoke_color=wheel_spoke_color
      link override Wheel Graphic: GraphicDiffuseColor=[0.2 0.2 0.2]
      settings: SourceProductBaseCode=MS
  Wheel 9 : sm_bumper_car_lib/Wheel  r=wheel_radius  rin=wheel_inner_radius  spoke_r=wheel_spoke_thickness  W=wheel_width  m=wheel_m  color=wheel_color  spoke_color=wheel_spoke_color
      link override Wheel Graphic: GraphicDiffuseColor=[0.2 0.2 0.2]
      settings: SourceProductBaseCode=MS
  R : PMIOPort  Side=Left
  Geom : PMIOPort  Port=2  Side=Right
  wires:
  In Bus Element3/1 -> Simulink-PS Converter3/1
  In Bus Element1/1 -> Simulink-PS Converter1/1
  In Bus Element5/1 -> Simulink-PS Converter6/1
  In Bus Element6/1 -> Simulink-PS Converter4/1
  In Bus Element4/1 -> Simulink-PS Converter5/1
  In Bus Element/1 -> Simulink-PS Converter7/1
  In Bus Element9/1 -> Simulink-PS Converter8/1
  In Bus Element2/1 -> Simulink-PS Converter2/1
  PS-Simulink Converter/1 -> Square/1
  PS-Simulink Converter1/1 -> Square1/1
  PS-Simulink Converter2/1 -> Square2/1
  PS-Simulink Converter3/1 -> Square3/1
  PS-Simulink Converter4/1 -> Square4/1
  PS-Simulink Converter5/1 -> Square5/1
  PS-Simulink Converter6/1 -> Square6/1
  PS-Simulink Converter7/1 -> Square7/1
  Square/1 -> Add/1
  Square1/1 -> Add/2
  Square2/1 -> Add/3
  Square3/1 -> Add/4
  Square4/1 -> Add/5
  Square5/1 -> Add/6
  Square6/1 -> Add/7
  Square7/1 -> Add/8
  Add/1 -> Scope/1, To Workspace/1
  connections:
  ToJoint/LConn1 -- Towheel1/LConn1 -- Link 1/RConn1 -- R/RConn1
  Towheel1/RConn1 -- Revolute Joint18/LConn1
  Wheel 4/LConn1 -- Revolute Joint5/RConn1
  Wheel 1/LConn1 -- Revolute Joint18/RConn1
  Simscape Bus/RConn1 -- Geom/RConn1
  Simscape Bus/LConn14 -- Link 1/LConn1
  Wheel 3/RConn1 -- Simscape Bus/LConn13
  Wheel 1/RConn1 -- Simscape Bus/LConn12
  Wheel 4/RConn1 -- Simscape Bus/LConn15
  Wheel 2/RConn1 -- Simscape Bus/LConn18
  ToLink/RConn1 -- Link 2/RConn1 -- ToJoint1/LConn1 -- Towheel2/LConn1
  Revolute Joint2/LConn1 -- ToJoint/RConn1
  ToLink/LConn1 -- Revolute Joint2/RConn1
  Simulink-PS Converter2/RConn1 -- Revolute Joint2/LConn2
  Revolute Joint1/LConn1 -- Towheel2/RConn1
  Wheel 2/LConn1 -- Revolute Joint1/RConn1
  ToLink1/LConn1 -- Revolute Joint4/RConn1
  Revolute Joint4/LConn1 -- ToJoint1/RConn1
  Towheel3/LConn1 -- ToJoint2/LConn1 -- ToLink1/RConn1 -- Link 3/RConn1
  Revolute Joint3/LConn1 -- Towheel3/RConn1
  Wheel 3/LConn1 -- Revolute Joint3/RConn1
  Towheel4/LConn1 -- ToJoint3/LConn1 -- Link 4/RConn1 -- ToLink2/RConn1
  ToLink2/LConn1 -- Revolute Joint6/RConn1
  Revolute Joint5/LConn1 -- Towheel4/RConn1
  Revolute Joint6/LConn1 -- ToJoint2/RConn1
  Simulink-PS Converter3/RConn1 -- Revolute Joint4/LConn2
  Revolute Joint6/LConn2 -- Simulink-PS Converter1/RConn1
  Link 2/LConn1 -- Simscape Bus/LConn9
  Link 3/LConn1 -- Simscape Bus/LConn10
  Link 4/LConn1 -- Simscape Bus/LConn11
  Towheel7/LConn1 -- ToJoint6/LConn1 -- ToLink5/RConn1 -- Link 7/RConn1
  ToLink3/RConn1 -- Link 5/RConn1 -- ToJoint4/LConn1 -- Towheel5/LConn1
  Towheel6/LConn1 -- Link 6/RConn1 -- ToJoint5/LConn1 -- ToLink4/RConn1
  ToLink4/LConn1 -- Revolute Joint10/RConn1
  Wheel 5/LConn1 -- Revolute Joint9/RConn1
  Revolute Joint11/LConn1 -- Towheel7/RConn1
  Revolute Joint9/LConn1 -- Towheel5/RConn1
  Simulink-PS Converter6/RConn1 -- Revolute Joint10/LConn2
  Revolute Joint10/LConn1 -- ToJoint4/RConn1
  Revolute Joint12/LConn1 -- ToJoint5/RConn1
  Revolute Joint7/LConn1 -- Towheel6/RConn1
  ToLink5/LConn1 -- Revolute Joint12/RConn1
  Wheel 7/LConn1 -- Revolute Joint11/RConn1
  ToLink3/LConn1 -- Revolute Joint8/RConn1
  Revolute Joint12/LConn2 -- Simulink-PS Converter4/RConn1
  Wheel 6/LConn1 -- Revolute Joint7/RConn1
  Simulink-PS Converter5/RConn1 -- Revolute Joint8/LConn2
  Revolute Joint8/LConn1 -- ToJoint3/RConn1
  Simscape Bus/LConn5 -- Wheel 6/RConn1
  Simscape Bus/LConn6 -- Link 7/LConn1
  Simscape Bus/LConn7 -- Wheel 5/RConn1
  Simscape Bus/LConn8 -- Wheel 7/RConn1
  Simscape Bus/LConn16 -- Link 5/LConn1
  Simscape Bus/LConn17 -- Link 6/LConn1
  Link 8/RConn1 -- Towheel8/LConn1 -- ToJoint7/LConn1 -- ToLink6/RConn1
  ToLink6/LConn1 -- Revolute Joint14/RConn1
  Revolute Joint14/LConn1 -- ToJoint6/RConn1
  Revolute Joint14/LConn2 -- Simulink-PS Converter7/RConn1
  Wheel 8/LConn1 -- Revolute Joint13/RConn1
  Revolute Joint13/LConn1 -- Towheel8/RConn1
  ToLink7/LConn1 -- Revolute Joint16/RConn1
  Revolute Joint16/LConn2 -- Simulink-PS Converter8/RConn1
  Revolute Joint16/LConn1 -- ToJoint7/RConn1
  Link 9/RConn1 -- ToLink7/RConn1 -- Towheel9/LConn1
  Towheel9/RConn1 -- Revolute Joint15/LConn1
  Revolute Joint15/RConn1 -- Wheel 9/LConn1
  Wheel 8/RConn1 -- Simscape Bus/LConn1
  Simscape Bus/LConn2 -- Link 8/LConn1
  Link 9/LConn1 -- Simscape Bus/LConn4
  Simscape Bus/LConn3 -- Wheel 9/RConn1
  PS-Simulink Converter/LConn1 -- Revolute Joint2/RConn2
  Revolute Joint4/RConn2 -- PS-Simulink Converter1/LConn1
  Revolute Joint6/RConn2 -- PS-Simulink Converter2/LConn1
  Revolute Joint8/RConn2 -- PS-Simulink Converter3/LConn1
  Revolute Joint10/RConn2 -- PS-Simulink Converter4/LConn1
  Revolute Joint12/RConn2 -- PS-Simulink Converter5/LConn1
  Revolute Joint14/RConn2 -- PS-Simulink Converter6/LConn1
  Revolute Joint16/RConn2 -- PS-Simulink Converter7/LConn1

== system Linearhopf_squaretorque_0_5/Subsystem ==
  Brick Solid : sm_lib/Body Elements/Brick Solid  GraphicAmbientColor=[0.15 0.15 0.15 1.0]  BasedOnType=Density  BrickDimensions=[50 50 1]  BrickDimensionUnits=m  CenterOfMass=[0 0 0]  CenterOfMassUnits=m  GraphicDiffuseColor=[0.5 0.5 0.5]  Density=1000  DensityUnits=kg/m^3  DoExposeReferenceFrame=on  GraphicEmissiveColor=[0.0 0.0 0.0 1.0]  ExportEntireGeometry=on  SerializedFrames=<Frames/>  MarkerShape=Sphere  MarkerSize=10  GraphicType=FromGeometry  InertiaType=CalculateFromGeometry  Mass=1  MassUnits=kg  MomentsOfInertia=[1 1 1]  MomentsOfInertiaUnits=kg*m^2  GraphicOpacity=1.0  ProductsOfInertia=[0 0 0]  ProductsOfInertiaUnits=kg*m^2  GraphicShininess=75  GraphicSpecularColor=[0.5 0.5 0.5 1.0]  GraphicVisPropType=SimpleVisualProperties
  Brick Solid1 : PMIOPort  Side=Right
  Brick Solid2 : PMIOPort  Port=2  Side=Right
  connections:
  Brick Solid1/RConn1 -- Brick Solid/RConn1
  Brick Solid/LConn1 -- Brick Solid2/RConn1

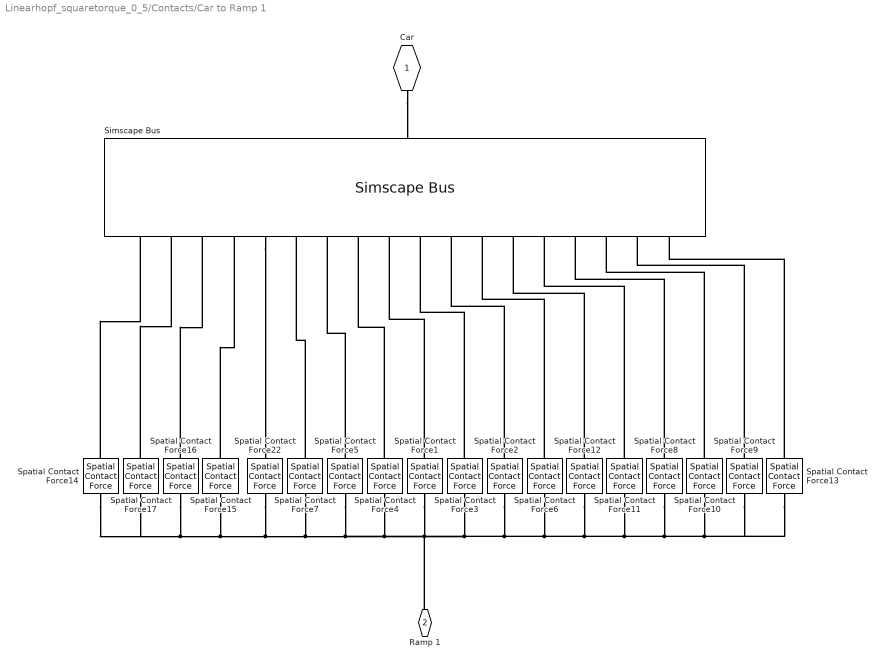
== system Linearhopf_squaretorque_0_5/Contacts/Car to Ramp 1 ==
  Simscape Bus : SimscapeBus  HierarchyStrings=Link8;Wheel8;Link9;Wheel9;Wheel6;Link7;Wheel5;Wheel7;Link2;Link3;Link4;BackLeft;FrontLeft;Link1;FrontRight;Link5;Link6;BackRight
  Spatial Contact Force{1..17,22} (18 alike) : sm_lib/Forces and Torques/Spatial Contact Force  CoefficientOfDynamicFriction=muk  CoefficientOfStaticFriction=mus  NormalDamping=b  NormalDampingUnits=N/(m/s)  NormalStiffness=k  NormalStiffnessUnits=N/m  FrictionalCriticalVelocity=cv  FrictionalCriticalVelocityUnits=m/s  SenseFrictionalForceMagnitude=off  SenseNormalForceMagnitude=off  SenseSeparationDistance=off  NormalTransitionRegionWidth=tau  NormalTransitionRegionWidthUnits=m  FrictionType=SmoothStickSlip
  Car : PMIOPort  Side=Right
  Ramp 1 : PMIOPort  Port=2  Side=Left
  connections:
  Spatial Contact Force13/LConn1 -- Spatial Contact Force9/LConn1 -- Spatial Contact Force10/LConn1 -- Spatial Contact Force8/LConn1 -- Spatial Contact Force11/LConn1 -- Spatial Contact Force12/LConn1 -- Spatial Contact Force6/LConn1 -- Spatial Contact Force2/LConn1 -- Ramp 1/RConn1 -- Spatial Contact Force14/LConn1 -- Spatial Contact Force17/LConn1 -- Spatial Contact Force16/LConn1 -- Spatial Contact Force15/LConn1 -- Spatial Contact Force22/LConn1 -- Spatial Contact Force7/LConn1 -- Spatial Contact Force5/LConn1 -- Spatial Contact Force4/LConn1 -- Spatial Contact Force1/LConn1 -- Spatial Contact Force3/LConn1
  Car/RConn1 -- Simscape Bus/RConn1
  Simscape Bus/LConn5 -- Spatial Contact Force22/RConn1
  Spatial Contact Force1/RConn1 -- Simscape Bus/LConn9
  Spatial Contact Force3/RConn1 -- Simscape Bus/LConn10
  Spatial Contact Force2/RConn1 -- Simscape Bus/LConn11
  Spatial Contact Force6/RConn1 -- Simscape Bus/LConn12
  Spatial Contact Force4/RConn1 -- Simscape Bus/LConn8
  Spatial Contact Force5/RConn1 -- Simscape Bus/LConn7
  Spatial Contact Force7/RConn1 -- Simscape Bus/LConn6
  Spatial Contact Force12/RConn1 -- Simscape Bus/LConn13
  Spatial Contact Force11/RConn1 -- Simscape Bus/LConn14
  Spatial Contact Force8/RConn1 -- Simscape Bus/LConn15
  Spatial Contact Force10/RConn1 -- Simscape Bus/LConn16
  Spatial Contact Force9/RConn1 -- Simscape Bus/LConn17
  Spatial Contact Force13/RConn1 -- Simscape Bus/LConn18
  Spatial Contact Force16/RConn1 -- Simscape Bus/LConn3
  Spatial Contact Force15/RConn1 -- Simscape Bus/LConn4
  Spatial Contact Force17/RConn1 -- Simscape Bus/LConn2
  Spatial Contact Force14/RConn1 -- Simscape Bus/LConn1
